simulink model "Model_3a_NH3_constant_clean"  (R2019a)
settings: Solver=FixedStepAuto  StartTime=0.0  StopTime=8760  FixedStep=1  RelTol=1e-3
libraries: simulink x7
settings Model: Creator=senja  LastModifiedBy=senja

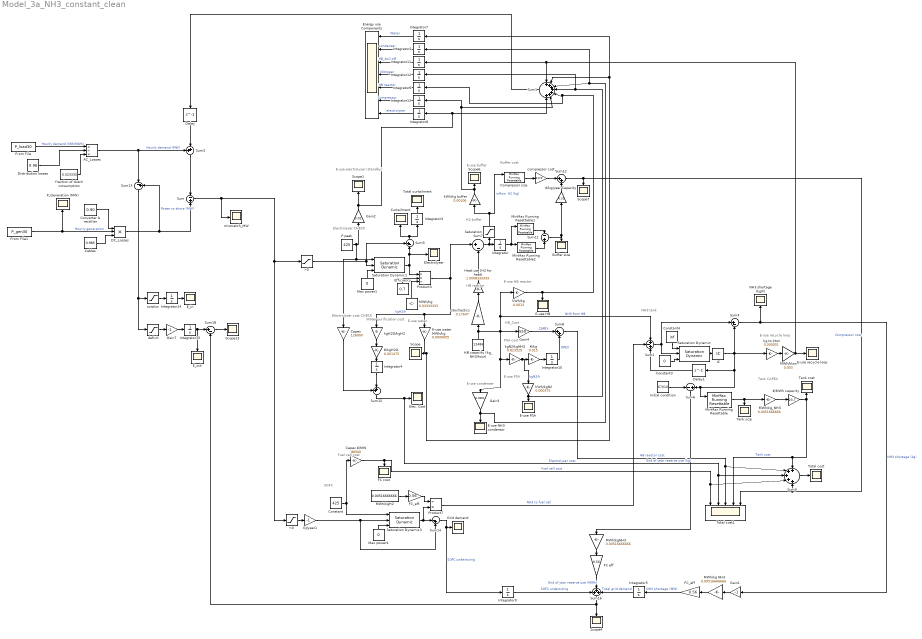
== system Model_3a_NH3_constant_clean ==
  note: PSA cost
  note: Water purification cost
  note: E-use buffer
  note: Buffer cost
  note: E-use HB reactor
  note: E-use PSA
  note: HB_Cost
  note: Tank CAPEX
  note: E-use recycle loop
  note: E-use condenser
  note: NH3 tank
  note: HB reactor
  note: E-use electrolyser (standby)
  note: E-use water
  note: Fuel cell cost
  note: SOFC
  note: Electrolyser CHECK
  note: Electrolyzer cost CHECK
  note: H2 buffer
  " Heat use (H2 for heat)" : Gain  Gain=1.0008333333
  <0 : Saturate  UpperLimit=0  LowerLimit=-inf
  >0 : Saturate
  AC_Losses : Product  Inputs=*/*
  Buffer size : Scope
  Cables : Constant  Value=0.985
  Capex : Gain  Gain=126000
  Capex €/MW : Gain  Gain=88500
  Compressor size : simulink/Math Operations/MinMax Running Resettable  Function=max  vinit=0.0
  Constant : Constant  Value=425
  Constant3 : Constant  Value=0
  Constant4 : Constant  Value=inf
  Converter & rectifier : Constant  Value=0.90
  Curtailment : Scope
  DC_Losses : Product  Inputs=3
  Delay : Delay  DelayLength=1  InitialCondition=0
  Delay1 : Delay  DelayLength=1
  Distribution losses : Constant  Value=0.96
  E-use HB : Scope
  E-use NH3 condensor : Scope
  E-use PSA : Scope
  E-use recycle loop : Scope
  E-use water MWh/kg : Gain  Gain=0.0000005
  E_in : Scope
  E_out : Scope
  Efficiency : Constant  Value=0.7
  Elec. Cost : Scope
  Electrolyser : Scope
  Energy use Components : Scope  NumInputPorts=7
  FC cost : Scope
  FC eff : Gain  Gain=0.56
  FC_eff : Gain  Gain=0.56
  FC_eff. : Gain  Gain=0.56
  From File : FromFile  FileName=P_load30  SampleTime=0
  From File1 : FromFile  FileName=P_gen30  SampleTime=0
  GJ/year1 : Gain  Gain=-1
  Gain1 : Gain  Gain=-1
  Gain2 : Gain  Gain=0.02
  Gain3 : Gain  Gain=0.0001
  Gain4 : Gain  Gain=550
  Gain7 : Gain  Gain=-1
  Grid demand : Scope
  HB capacity (kg_NH3/hour) : Constant  Value=12486
  IC : InitialCondition  Value=67010
  Initial condition : Constant  Value=67010
  Integrator{,2..15} (15 alike) : Integrator
  MWh/kg : Constant  Value=0.03333333
  MWh/kg NH3 : Gain  Gain=0.00516666666
  MWh/kgH2 : Constant  Value=0.00516666666
  "MWh/kgNH3 " : Gain  Gain=0.00516666666
  MWh/kg_NH3 : Gain  Gain=0.0051666666
  MWh/kton : Gain  Gain=0.003
  Max power1 : Constant  Value=0
  Max power4 : Constant  Value=0
  MinMax Running Resettable : simulink/Math Operations/MinMax Running Resettable  Function=max  vinit=0.0
  MinMax Running Resettable1 : simulink/Math Operations/MinMax Running Resettable  Function=min  vinit=0.0
  MinMax Running Resettable2 : simulink/Math Operations/MinMax Running Resettable  Function=max  vinit=0.0
  NH3 shortage (kg/h) : Scope
  P peek : Constant  Value=425
  P_Generation (MW) : Scope
  Product3 : Product  Inputs=**/
  Product7 : Product  Inputs=/*
  Saturation : Saturate  UpperLimit=inf  LowerLimit=0
  Saturation Dynamic : simulink/Discontinuities/Saturation Dynamic  OutMin=[]  OutMax=[]  OutDataTypeStr=Inherit: Same as second input  OutDataType=fixdt(1, 16)  OutScaling=2^-10  DoSatur=off
  Saturation Dynamic1 : simulink/Discontinuities/Saturation Dynamic  OutMin=[]  OutMax=[]  OutDataTypeStr=Inherit: Same as second input  OutDataType=fixdt(1, 16)  OutScaling=2^-10  DoSatur=off
  Saturation Dynamic3 : simulink/Discontinuities/Saturation Dynamic  OutMin=[]  OutMax=[]  OutDataTypeStr=Inherit: Same as second input  OutDataType=fixdt(1, 16)  OutScaling=2^-10  DoSatur=off
  Scope{,1,4,6..7,13} (6 alike) : Scope
  Sum : Sum  Inputs=-|+
  Sum1 : Sum  Inputs=+++++++
  Sum11 : Sum  Inputs=-|+
  Sum12 : Sum  Inputs=|++
  Sum13 : Sum  Inputs=|-+
  Sum14 : Sum  Inputs=|-+
  Sum15 : Sum  Inputs=++|
  Sum16 : Sum  Inputs=+++
  Sum18 : Sum  Inputs=|+-
  Sum2 : Sum  Inputs=+-+
  Sum3 : Sum  Inputs=++|
  Sum4 : Sum  Inputs=|+-
  Sum5 : Sum  Inputs=+-|
  Sum6 : Sum  Inputs=-|+
  Sum7 : Sum  Inputs=|+-
  Sum8 : Sum  Inputs=|++
  Sum9 : Sum  Inputs=+++++
  Tank cost : Scope
  Tank size : Scope
  Total cost : Scope
  Total cost1 : Scope  NumInputPorts=5
  Total curtailment : Scope
  compressor cost : Gain  Gain=1170
  deficit : Saturate  UpperLimit=0  LowerLimit=-inf
  fraction of dutch consumption : Constant  Value=0.023335
  kWh/kg : Gain  Gain=0.0013
  kWh/kg buffer : Gain  Gain=0.00106
  kWh/kgN2 : Gain  Gain=0.000375
  kg to kton : Gain  Gain=0.000001
  kgH2O/kgH2 : Gain  Gain=9
  kgN2/kgNH3 : Gain  Gain=0.823529
  mismatch_MW : Scope
  stochastics : Gain  Gain=0.17647
  surplus : Saturate  UpperLimit=inf  LowerLimit=0
  €/MWh capacity : Gain  Gain=23.7
  €/kg : Gain  Gain=0.015
  €/kg/year Capacity : Gain  Gain=0.31
  €/kgH2O : Gain  Gain=0.001375
  wires:
  From File/1 -> AC_Losses/1  "Hourly demand (MW/MWh)"
  Efficiency/1 -> Product3/2
  fraction of dutch consumption/1 -> AC_Losses/3
  Distribution losses/1 -> AC_Losses/2
  Cables/1 -> DC_Losses/3
  Converter & rectifier/1 -> DC_Losses/1
  DC_Losses/1 -> Sum13/2, Sum/2  "Power to shore (MW)"
  >0/1 -> Saturation Dynamic1/2, Sum5/1
  <0/1 -> GJ/year1/1
  AC_Losses/1 -> Sum3/1, Sum13/1  "Hourly demand (MW)"
  From File1/1 -> P_Generation (MW)/1, DC_Losses/2  "Hourly generation"
  Max power1/1 -> Saturation Dynamic1/3
  Saturation Dynamic1/1 -> Sum5/2, Electrolyser/1, Product3/1
  Capex/1 -> Sum15/1
  Sum15/1 -> Sum9/3, Total cost1/2, Elec. Cost/1  "Electrolyser cost"
  €/kgH2O/1 -> Integrator4/1
  P peek/1 -> Saturation Dynamic1/1, Capex/1, Gain2/1
  GJ/year1/1 -> Sum14/2, Saturation Dynamic3/2
  Product3/1 -> E-use water MWh/kg/1, kgH2O/kgH2/1, Sum7/1  "kgH2/h"
  Sum/1 -> <0/1, >0/1, mismatch_MW/1
  Sum9/1 -> Total cost/1
  Constant/1 -> Saturation Dynamic3/1, Capex €/MW/1
  Max power4/1 -> Saturation Dynamic3/3
  Saturation Dynamic3/1 -> Sum14/1, Product7/2
  MWh/kgH2/1 -> FC_eff./1
  Integrator3/1 -> Total curtailment/1
  kgH2O/kgH2/1 -> €/kgH2O/1
  Integrator4/1 -> Sum15/2
  MWh/kg/1 -> Product3/3
  Capex €/MW/1 -> FC cost/1, Total cost1/1, Sum9/4  "Fuel cell cost"
  FC_eff./1 -> Product7/1
  Sum5/1 -> Integrator3/1, Curtailment/1
  Sum14/1 -> Integrator9/1, Grid demand/1  "SOFC undersizing"
  E-use water MWh/kg/1 -> Sum1/2, Integrator7/1, Scope/1
  Gain2/1 -> Scope1/1, Sum1/7, Integrator8/1
  Sum3/1 -> Sum/1
  Sum1/1 -> Delay/1
  Delay/1 -> Sum3/2
  Integrator2/1 -> Energy use Components/2  "condenser"
  Integrator6/1 -> Energy use Components/5  "HB reactor"
  Integrator7/1 -> Energy use Components/1  "Water"
  Integrator8/1 -> Energy use Components/7  "electrolyser"
  Product7/1 -> Sum2/2  "NH3 to fuel cell"
  Sum7/1 -> Saturation/1, Integrator/1
  Integrator/1 -> MinMax Running Resettable1/1, MinMax Running Resettable2/1
  stochastics/1 -> " Heat use (H2 for heat)"/1
  HB capacity (kg_NH3/hour)/1 -> Gain3/1, kgN2/kgNH3/1, Sum2/1, kWh/kg/1, Gain4/1, stochastics/1  "NH3 from HB"
  Sum2/1 -> Sum4/1, Saturation Dynamic/2
  Delay1/1 -> Sum2/3
  Constant3/1 -> Saturation Dynamic/3
  Sum4/1 -> Gain1/1, NH3 shortage (kg/h)/1  "NH3 shortage (kg)"
  MWh/kg NH3/1 -> FC_eff/1
  FC_eff/1 -> Integrator5/1  "NH3 shortage (MW)"
  Saturation Dynamic/1 -> IC/1
  IC/1 -> Sum4/2, kg to kton/1, Sum6/2, MinMax Running Resettable/1, Delay1/1
  Initial condition/1 -> Sum6/1
  "MWh/kgNH3 "/1 -> FC eff/1
  FC eff/1 -> Sum16/2  "End of year reserve use (MWh)"
  Sum6/1 -> "MWh/kgNH3 "/1  "End of year reserve use (kg)"
  Gain1/1 -> MWh/kg NH3/1
  Integrator9/1 -> Sum16/1  "SOFC undersizing"
  Constant4/1 -> Saturation Dynamic/1
  Gain3/1 -> E-use NH3 condensor/1, Integrator2/1, Sum1/3
  MWh/kton/1 -> E-use recycle loop/1, Sum1/1, Integrator11/1
  kg to kton/1 -> MWh/kton/1
  MWh/kg_NH3/1 -> €/MWh capacity/1
  €/MWh capacity/1 -> Total cost1/4, Sum9/1, Tank cost/1  "Tank cost"
  Gain4/1 -> Sum8/1  "CAPEX"
  kgN2/kgNH3/1 -> kWh/kgN2/1, €/kg/1  "kgN2/h"
  €/kg/1 -> Integrator10/1
  Sum8/1 -> Sum9/2, Total cost1/3  "HB reactor cost"
  Integrator10/1 -> Sum8/2  "OPEX"
  " Heat use (H2 for heat)"/1 -> Sum7/2
  kWh/kg/1 -> Sum1/5, Integrator6/1, E-use HB/1
  Integrator12/1 -> Energy use Components/4  "Nitrogen"
  Integrator11/1 -> Energy use Components/3  "HB_boil off"
  kWh/kgN2/1 -> Integrator12/1, Sum1/4, E-use PSA/1
  MinMax Running Resettable1/1 -> Sum11/1
  MinMax Running Resettable2/1 -> Sum11/2
  Sum11/1 -> €/kg/year Capacity/1, Buffer size/1
  €/kg/year Capacity/1 -> Sum12/2
  kWh/kg buffer/1 -> Integrator13/1, Sum1/6, Scope6/1
  Saturation/1 -> Compressor size/1, kWh/kg buffer/1  "inflow  H2 (kg)"
  Compressor size/1 -> compressor cost/1
  compressor cost/1 -> Sum12/1
  Sum12/1 -> Total cost1/5, Sum9/5, Scope7/1  "Compressor cost"
  Integrator13/1 -> Energy use Components/6  "Compressor"
  deficit/1 -> Gain7/1
  Sum13/1 -> surplus/1, deficit/1
  Gain7/1 -> Integrator15/1
  Sum18/1 -> Scope13/1
  Integrator14/1 -> E_in/1
  surplus/1 -> Integrator14/1
  Integrator15/1 -> Sum18/1, E_out/1
  Sum16/1 -> Scope4/1, Sum18/2
  MinMax Running Resettable/1 -> Tank size/1, MWh/kg_NH3/1
  Integrator5/1 -> Sum16/3  "Total grid demand"
